simulink model "HVPS120PFC_sfun"  (R2022b)
settings: configuration reference "ModelConfig_var" (kept outside this file)
undefined symbols (not defined in the file or in its folder): InputCircuit
libraries: HVPS_AC120V_PFC_sfun_xk x1
settings Model: Creator=KIRTACA  LastModifiedBy=BEDNASA
settings ConfigSetRef: SourceName=ModelConfig_var  SourceLocation=Base Workspace

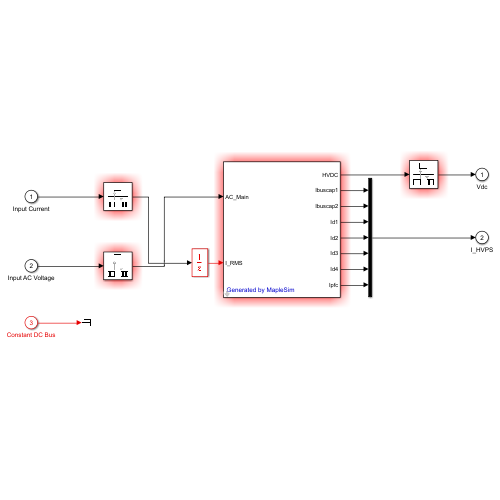
[thumbnail: Simulink's stored preview of the top-level diagram]
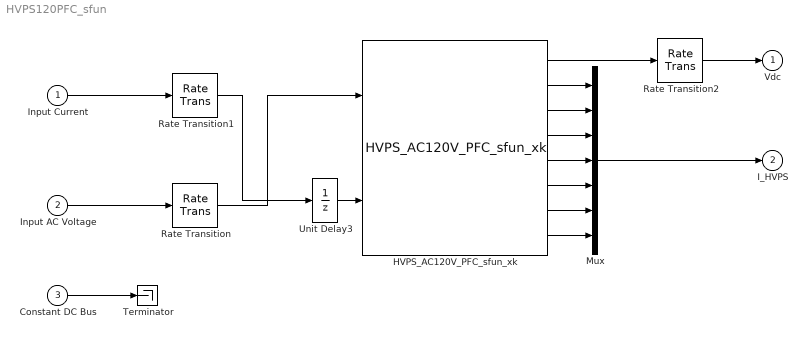
== system HVPS120PFC_sfun ==
  Input Current : Inport
  Input AC Voltage : Inport  Port=2
  Constant DC Bus : Inport  Port=3
  HVPS_AC120V_PFC_sfun_xk : HVPS_AC120V_PFC_sfun_xk/HVPS_AC120V_PFC_sfun_xk  Description=Subsystem: HVPS_AC120V_PFC_sfun_xk  ic=[InputCircuit.Vr*sqrt(2), InputCircuit.Vr*sqrt(2), 0.]  Par1=InputCircuit.C_buscap  Par2=InputCircuit.G_off  Par3=InputCircuit.L_line  Par4=InputCircuit.L_pfc  Par5=InputCircuit.R_buscap  Par6=InputCircuit.R_diode  Par7=InputCircuit.R_line  Par8=InputCircuit.R_pfc  Par9=298.15  Par10=0.  Par11=298.15  Par12=0.  Par13=298.15  Par14=0.  Par15=298.15  Par16=0.  Par17=.1e-1  Par18=298.15  Par19=298.15  Par20=.1e8  Par21=298.15  Par22=298.15  Par23=298.15  Par24=298.15  Par25=.4041e-2  Par26=298.15  Par27=298.15  Par28=.4041e-2  Par29=298.15  Par30=298.15  Par31=298.15  Par32=298.15  Par33=.4041e-2  Par34=1.  Par35=1.  Par36=.3e-2  Par37=.1e4  Par38=TimeSteps.ModelStep  MinStep=1/40  TimeStep_Solver=TimeSteps.ModelStep
  Mux : Mux  Inputs=7
  Rate Transition : RateTransition  InitialCondition=InputCircuit.Vr  OutPortSampleTime=TimeSteps.InputCircuitStep
  Rate Transition1 : RateTransition  OutPortSampleTime=TimeSteps.InputCircuitStep
  Rate Transition2 : RateTransition  InitialCondition=InputCircuit.Vdc_i  OutPortSampleTime=TimeSteps.ModelStep
  Terminator : Terminator
  Unit Delay3 : UnitDelay  SampleTime=-1  HasFrameUpgradeWarning=on
  Vdc : Outport  VectorParamsAs1DForOutWhenUnconnected=off
  I_HVPS : Outport  Port=2  VectorParamsAs1DForOutWhenUnconnected=off
  wires:
  Input AC Voltage/1 -> Rate Transition/1
  Input Current/1 -> Rate Transition1/1
  Rate Transition2/1 -> Vdc/1
  Constant DC Bus/1 -> Terminator/1
  HVPS_AC120V_PFC_sfun_xk/1 -> Rate Transition2/1
  Rate Transition/1 -> HVPS_AC120V_PFC_sfun_xk/1
  Unit Delay3/1 -> HVPS_AC120V_PFC_sfun_xk/2
  Rate Transition1/1 -> Unit Delay3/1
  Mux/1 -> I_HVPS/1
  HVPS_AC120V_PFC_sfun_xk/2 -> Mux/1
  HVPS_AC120V_PFC_sfun_xk/3 -> Mux/2
  HVPS_AC120V_PFC_sfun_xk/4 -> Mux/3
  HVPS_AC120V_PFC_sfun_xk/5 -> Mux/4
  HVPS_AC120V_PFC_sfun_xk/6 -> Mux/5
  HVPS_AC120V_PFC_sfun_xk/7 -> Mux/6
  HVPS_AC120V_PFC_sfun_xk/8 -> Mux/7
